simulink model "data"  (R2024b)
settings: Solver=ode4  StartTime=0.0  StopTime=simulation_time  FixedStep=sample_time  RelTol=1e-3
values from neighbouring files (symbols this model uses):
  init_dq = initial(i).init_dq    [LyaOrder8.m]
  init_q = initial(i).init_q    [LyaOrder8.m]
settings Model: Creator=zhes  LastModifiedBy=zhes

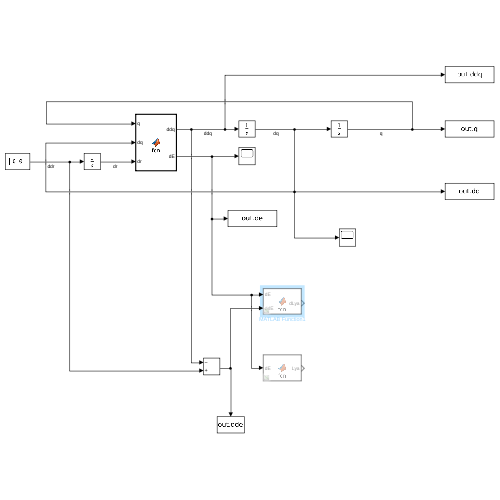
[thumbnail: Simulink's stored preview of the top-level diagram]
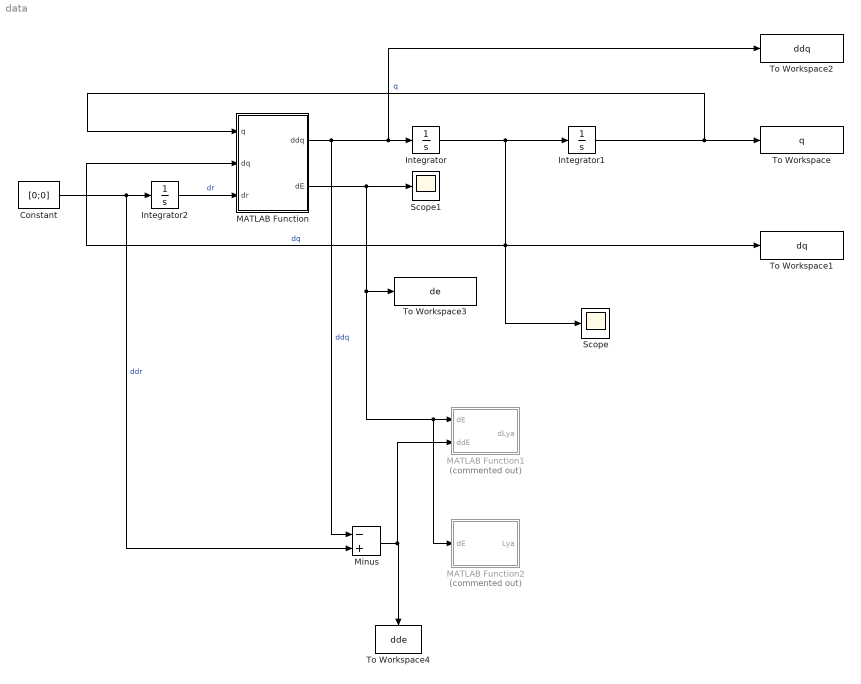
== system data ==
  Constant : Constant  Value=[0;0]
  Integrator : Integrator  InitialCondition=init_dq
  Integrator1 : Integrator  InitialCondition=init_q
  Integrator2 : Integrator  InitialCondition=[ 1 ; 1 ]
  MATLAB Function : MATLAB Function  TreatAsAtomicUnit=on
  MATLAB Function1 : MATLAB Function  Commented=on  TreatAsAtomicUnit=on
  MATLAB Function2 : MATLAB Function  Commented=on  TreatAsAtomicUnit=on
  Minus : Sum  Inputs=-+
  Scope : Scope
  Scope1 : Scope
  To Workspace : ToWorkspace  VariableName=q  SaveFormat=Structure With Time  SampleTime=-1
  To Workspace1 : ToWorkspace  VariableName=dq  SaveFormat=Structure With Time  SampleTime=-1
  To Workspace2 : ToWorkspace  VariableName=ddq  SaveFormat=Structure With Time  SampleTime=-1
  To Workspace3 : ToWorkspace  VariableName=de  SaveFormat=Structure With Time  SampleTime=-1
  To Workspace4 : ToWorkspace  VariableName=dde  SaveFormat=Structure With Time  SampleTime=-1
  wires:
  Integrator/1 -> MATLAB Function/2(dq), To Workspace1/1, Scope/1, Integrator1/1  "dq"
  Integrator1/1 -> To Workspace/1, MATLAB Function/1(q)  "q"
  MATLAB Function/1(ddq) -> Minus/1, To Workspace2/1, Integrator/1  "ddq"
  Integrator2/1 -> MATLAB Function/3(dr)  "dr"
  MATLAB Function/2(dE) -> MATLAB Function2/1(dE), MATLAB Function1/1(dE), To Workspace3/1, Scope1/1
  Constant/1 -> Minus/2, Integrator2/1  "ddr"
  Minus/1 -> MATLAB Function1/2(ddE), To Workspace4/1

== matlab function data/MATLAB Function1 ==
  data: dE input; dLya output; ddE input
function dLya = fcn(dE, ddE)

de1 = dE(1);
de2 = dE(2);

dde1 = ddE(1);
dde2 = ddE(2);

A = eye(2);

== matlab function data/MATLAB Function ==
  data: q input; ddq output; dq input; dr input; dE output
function [ddq, dE]= fcn(q, dq, dr)

q1 = q(1);
q2 = q(2);
dq1 = dq(1);
dq2 = dq(2);

dr1 = dr(1);
dr2 = dr(2);

kD = diag([10,10]);

de1 = dr1 - dq1;
de2 = dr2 - dq2;

dE = [de1; de2];

ddq = kD * dE;

== matlab function data/MATLAB Function2 ==
  data: dE input; Lya output
function Lya = fcn(dE)

de1 = dE(1);
de2 = dE(2);

A = eye(2);

Lya =
